simulink model "quadcopter_dyn_1"  (R2021b)
settings: Solver=VariableStepAuto  StartTime=0.0  StopTime=10.0  RelTol=1e-3
values from neighbouring files (symbols this model uses):
  g = 9.81    [quadcopter_dyn_1_param.m]
  J1 = 1    [quadcopter_dyn_1_param.m]
  J2 = 1    [quadcopter_dyn_1_param.m]
  J3 = 1    [quadcopter_dyn_1_param.m]
  l = 1    [quadcopter_dyn_1_param.m]
  m = 1    [quadcopter_dyn_1_param.m]
  rho = 1    [quadcopter_dyn_1_param.m]
settings Model: Creator=Chuong  LastModifiedBy=Chuong

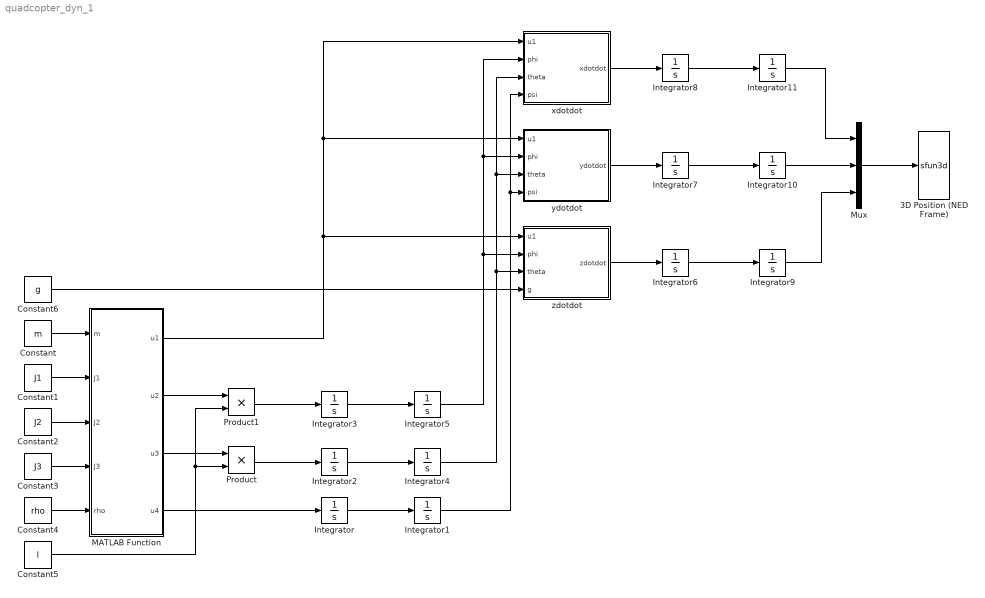
== system quadcopter_dyn_1 ==
  3D Position (NED Frame) : S-Function  LoadFcn=if exist('sfun3d','file'), sfun3d([],[],[],'LoadBlock'); end  FunctionName=sfun3d  Parameters=ax,T,np,cp,gd,ls,mk,mx,hd,tb  SFunctionDeploymentMode=off  EnableBusSupport=off  mask(3D Graph){np=1, ax=[-10 10 -10 10 -10 10], mx=1e4, T=0.1, cp=[9 6 3], gd=on, hd=off, tb=off, ls=-, mk=none}
      mask prompts: np "Number of moving points (lines)"; ax "Range: [xmin xmax  ymin ymax zmin zmax]"; mx "Max number of points in each line"; T "Sampling Time"; cp "Camera position (use [0 0 1] for 2D XY view)"; gd "Grid (on|off)"; hd "HeadMarkers (on|off)"; tb "Toolbar (on|off)"; ls "LineStyle"; mk "LineMarker"
      mask help:
      | This block plots the position of several points in the XYZ space. The input contains the coordinates of all the points (x1,y1,z1,x2,y2,z2,...).
      | The number of moving points (lines), the XYZ ranges, sampling time, camera position, and grid (among other things) can be set as mask parameters.
      settings: CopyFcn=if exist('sfun3d','file'), sfun3d([],[],[],'CopyBlock'); end  DeleteFcn=if exist('sfun3d','file'), sfun3d([],[],[],'DeleteBlock'); end  NameChangeFcn=if exist('sfun3d','file'), sfun3d([],[],[],'NameChange'); end
      mask Help:
      | This block plots the position of several points in the XYZ space. The input contains the coordinates of all the points (x1,y1,z1,x2,y2,z2,...).
      | The number of moving points (lines), the XYZ ranges, sampling time, camera position, and grid (among other things) can be set as mask parameters.
      mask TypeOptions ls: - | -- | : | -. | none
      mask TypeOptions mk: none | . | + | o | * | x | square | diamond | v | ^ | > | < | pentagram | hexagram
      mask Display: plot([.05 .95 .95 .05 .05],[.45 .45 .95 .95 .45], 0.5+cos(0:0.1:2*pi)*0.3,0.7+sin(0:0.1:2*pi)*0.2)
  Constant : Constant  Value=m
  Constant1 : Constant  Value=J1
  Constant2 : Constant  Value=J2
  Constant3 : Constant  Value=J3
  Constant4 : Constant  Value=rho
  Constant5 : Constant  Value=l
  Constant6 : Constant  Value=g
  Integrator{,1..11} (12 alike) : Integrator
  MATLAB Function : MATLAB Function  TreatAsAtomicUnit=on
  Mux : Mux  Inputs=3
  Product : Product
  Product1 : Product
  xdotdot : MATLAB Function  TreatAsAtomicUnit=on
  ydotdot : MATLAB Function  TreatAsAtomicUnit=on
  zdotdot : MATLAB Function  TreatAsAtomicUnit=on
  wires:
  Constant/1 -> MATLAB Function/1(m)
  Constant1/1 -> MATLAB Function/2(J1)
  Constant2/1 -> MATLAB Function/3(J2)
  Constant3/1 -> MATLAB Function/4(J3)
  Constant4/1 -> MATLAB Function/5(rho)
  MATLAB Function/4(u4) -> Integrator/1
  Integrator/1 -> Integrator1/1
  MATLAB Function/3(u3) -> Product/1
  Constant5/1 -> Product1/2, Product/2
  MATLAB Function/2(u2) -> Product1/1
  Product/1 -> Integrator2/1
  Product1/1 -> Integrator3/1
  Integrator2/1 -> Integrator4/1
  Integrator3/1 -> Integrator5/1
  Integrator5/1 -> zdotdot/2(phi), xdotdot/2(phi), ydotdot/2(phi)
  Integrator4/1 -> xdotdot/3(theta), ydotdot/3(theta), zdotdot/3(theta)
  Integrator1/1 -> xdotdot/4(psi), ydotdot/4(psi)
  MATLAB Function/1(u1) -> zdotdot/1(u1), ydotdot/1(u1), xdotdot/1(u1)
  Constant6/1 -> zdotdot/4(g)
  zdotdot/1(zdotdot) -> Integrator6/1
  ydotdot/1(ydotdot) -> Integrator7/1
  xdotdot/1(xdotdot) -> Integrator8/1
  Integrator6/1 -> Integrator9/1
  Integrator7/1 -> Integrator10/1
  Integrator8/1 -> Integrator11/1
  Integrator11/1 -> Mux/1
  Integrator10/1 -> Mux/2
  Integrator9/1 -> Mux/3
  Mux/1 -> 3D Position (NED Frame)/1

== matlab function quadcopter_dyn_1/xdotdot ==
  data: u1 input; xdotdot output; phi input; theta input; psi input
function xdotdot  = fcn(u1,phi,theta,psi)

xdotdot = u1*(cos(phi)*sin(theta)*cos(psi)+sin(phi)*sin(psi));

== matlab function quadcopter_dyn_1/MATLAB Function ==
  data: m input; J1 input; J2 input; J3 input; rho input; u1 output; u2 output; u3 output; u4 output
function [u1,u2,u3,u4] = fcn(m,J1,J2,J3,rho)

% m = mass
% Ji = moment of inertia w.r.t each axis
% rho = force-to-moment scaling factor

F1 = 1;
F2 = 1;
F3 = 1;
F4 = 1;

% u1 normalized total lift force
% u2, u3 and u4 correspond to the control inputs of roll, pitch and yaw 
% moments, respectively.

u1 = (F1 + F2 + F3 + F4)/m;     % Normalized total lift force
u2 = (F2-F4)/J1;                % Roll
u3 = (-F1+F3)/J2;               % Pitch
u4 = rho*(F1-F2+F3-F4)/J3;      % Yaw

== matlab function quadcopter_dyn_1/ydotdot ==
  data: u1 input; ydotdot output; phi input; theta input; psi input
function ydotdot = fcn(u1,phi,theta,psi)

ydotdot = u1*(cos(phi)*sin(theta)*sin(psi)-sin(phi)*cos(psi));

== matlab function quadcopter_dyn_1/zdotdot ==
  data: u1 input; zdotdot output; phi input; theta input; g input
function zdotdot = fcn(u1,phi,theta,g)

zdotdot = u1*(cos(phi)*cos(theta))-g;
